simulink model "signal_tranmission"  (R2024b)
settings: Solver=ode45  StartTime=0.0  StopTime=10  FixedStep=0.000125  RelTol=1e-3
libraries: dspfdesign x500, commchan3 x1
(part 5 of 7)

== system signal_tranmission/SSB Demod55/Balanced Modulator1 ==
  note: -S2(t)
  note: S1(t)
  note: -m(t)
  note: m(t)
  note: S2(t)
  note: S1(t)
  Input Signal : Inport
  Carrier Signal : Inport  Port=2
  -S2(t) : Product
  Add : Sum
  Add1 : Sum
  Add2 : Sum
  Constant : Constant
  Constant1 : Constant  Value=-1
  Constant2 : Constant
  Constant3 : Constant  Value=-1
  Product1 : Product
  S1(t) : Product
  S2(t) : Product
  DSBSC : Outport
  wires:
  Product1/1 -> Add1/1
  Add/1 -> S1(t)/1
  Constant3/1 -> -S2(t)/2
  Constant2/1 -> Add1/2
  S2(t)/1 -> -S2(t)/1
  Carrier Signal/1 -> S1(t)/2, S2(t)/1
  Constant/1 -> Add/2
  Add1/1 -> S2(t)/2
  Constant1/1 -> Product1/2
  -S2(t)/1 -> Add2/2
  S1(t)/1 -> Add2/1
  Input Signal/1 -> Product1/1, Add/1
  Add2/1 -> DSBSC/1

== system signal_tranmission/SSB Demod56/Balanced Modulator1 ==
  note: -S2(t)
  note: S1(t)
  note: -m(t)
  note: m(t)
  note: S2(t)
  note: S1(t)
  Input Signal : Inport
  Carrier Signal : Inport  Port=2
  -S2(t) : Product
  Add : Sum
  Add1 : Sum
  Add2 : Sum
  Constant : Constant
  Constant1 : Constant  Value=-1
  Constant2 : Constant
  Constant3 : Constant  Value=-1
  Product1 : Product
  S1(t) : Product
  S2(t) : Product
  DSBSC : Outport
  wires:
  Product1/1 -> Add1/1
  Add/1 -> S1(t)/1
  Constant3/1 -> -S2(t)/2
  Constant2/1 -> Add1/2
  S2(t)/1 -> -S2(t)/1
  Carrier Signal/1 -> S1(t)/2, S2(t)/1
  Constant/1 -> Add/2
  Add1/1 -> S2(t)/2
  Constant1/1 -> Product1/2
  -S2(t)/1 -> Add2/2
  S1(t)/1 -> Add2/1
  Input Signal/1 -> Product1/1, Add/1
  Add2/1 -> DSBSC/1

== system signal_tranmission/SSB Demod57/Balanced Modulator1 ==
  note: -S2(t)
  note: S1(t)
  note: -m(t)
  note: m(t)
  note: S2(t)
  note: S1(t)
  Input Signal : Inport
  Carrier Signal : Inport  Port=2
  -S2(t) : Product
  Add : Sum
  Add1 : Sum
  Add2 : Sum
  Constant : Constant
  Constant1 : Constant  Value=-1
  Constant2 : Constant
  Constant3 : Constant  Value=-1
  Product1 : Product
  S1(t) : Product
  S2(t) : Product
  DSBSC : Outport
  wires:
  Product1/1 -> Add1/1
  Add/1 -> S1(t)/1
  Constant3/1 -> -S2(t)/2
  Constant2/1 -> Add1/2
  S2(t)/1 -> -S2(t)/1
  Carrier Signal/1 -> S1(t)/2, S2(t)/1
  Constant/1 -> Add/2
  Add1/1 -> S2(t)/2
  Constant1/1 -> Product1/2
  -S2(t)/1 -> Add2/2
  S1(t)/1 -> Add2/1
  Input Signal/1 -> Product1/1, Add/1
  Add2/1 -> DSBSC/1

== system signal_tranmission/SSB Demod58/Balanced Modulator1 ==
  note: -S2(t)
  note: S1(t)
  note: -m(t)
  note: m(t)
  note: S2(t)
  note: S1(t)
  Input Signal : Inport
  Carrier Signal : Inport  Port=2
  -S2(t) : Product
  Add : Sum
  Add1 : Sum
  Add2 : Sum
  Constant : Constant
  Constant1 : Constant  Value=-1
  Constant2 : Constant
  Constant3 : Constant  Value=-1
  Product1 : Product
  S1(t) : Product
  S2(t) : Product
  DSBSC : Outport
  wires:
  Product1/1 -> Add1/1
  Add/1 -> S1(t)/1
  Constant3/1 -> -S2(t)/2
  Constant2/1 -> Add1/2
  S2(t)/1 -> -S2(t)/1
  Carrier Signal/1 -> S1(t)/2, S2(t)/1
  Constant/1 -> Add/2
  Add1/1 -> S2(t)/2
  Constant1/1 -> Product1/2
  -S2(t)/1 -> Add2/2
  S1(t)/1 -> Add2/1
  Input Signal/1 -> Product1/1, Add/1
  Add2/1 -> DSBSC/1

== system signal_tranmission/SSB Demod59/Balanced Modulator1 ==
  note: -S2(t)
  note: S1(t)
  note: -m(t)
  note: m(t)
  note: S2(t)
  note: S1(t)
  Input Signal : Inport
  Carrier Signal : Inport  Port=2
  -S2(t) : Product
  Add : Sum
  Add1 : Sum
  Add2 : Sum
  Constant : Constant
  Constant1 : Constant  Value=-1
  Constant2 : Constant
  Constant3 : Constant  Value=-1
  Product1 : Product
  S1(t) : Product
  S2(t) : Product
  DSBSC : Outport
  wires:
  Product1/1 -> Add1/1
  Add/1 -> S1(t)/1
  Constant3/1 -> -S2(t)/2
  Constant2/1 -> Add1/2
  S2(t)/1 -> -S2(t)/1
  Carrier Signal/1 -> S1(t)/2, S2(t)/1
  Constant/1 -> Add/2
  Add1/1 -> S2(t)/2
  Constant1/1 -> Product1/2
  -S2(t)/1 -> Add2/2
  S1(t)/1 -> Add2/1
  Input Signal/1 -> Product1/1, Add/1
  Add2/1 -> DSBSC/1

== system signal_tranmission/SSB Demod6/Balanced Modulator1 ==
  note: -S2(t)
  note: S1(t)
  note: -m(t)
  note: m(t)
  note: S2(t)
  note: S1(t)
  Input Signal : Inport
  Carrier Signal : Inport  Port=2
  -S2(t) : Product
  Add : Sum
  Add1 : Sum
  Add2 : Sum
  Constant : Constant
  Constant1 : Constant  Value=-1
  Constant2 : Constant
  Constant3 : Constant  Value=-1
  Product1 : Product
  S1(t) : Product
  S2(t) : Product
  DSBSC : Outport
  wires:
  Product1/1 -> Add1/1
  Add/1 -> S1(t)/1
  Constant3/1 -> -S2(t)/2
  Constant2/1 -> Add1/2
  S2(t)/1 -> -S2(t)/1
  Carrier Signal/1 -> S1(t)/2, S2(t)/1
  Constant/1 -> Add/2
  Add1/1 -> S2(t)/2
  Constant1/1 -> Product1/2
  -S2(t)/1 -> Add2/2
  S1(t)/1 -> Add2/1
  Input Signal/1 -> Product1/1, Add/1
  Add2/1 -> DSBSC/1

== system signal_tranmission/SSB Demod60/Balanced Modulator1 ==
  note: -S2(t)
  note: S1(t)
  note: -m(t)
  note: m(t)
  note: S2(t)
  note: S1(t)
  Input Signal : Inport
  Carrier Signal : Inport  Port=2
  -S2(t) : Product
  Add : Sum
  Add1 : Sum
  Add2 : Sum
  Constant : Constant
  Constant1 : Constant  Value=-1
  Constant2 : Constant
  Constant3 : Constant  Value=-1
  Product1 : Product
  S1(t) : Product
  S2(t) : Product
  DSBSC : Outport
  wires:
  Product1/1 -> Add1/1
  Add/1 -> S1(t)/1
  Constant3/1 -> -S2(t)/2
  Constant2/1 -> Add1/2
  S2(t)/1 -> -S2(t)/1
  Carrier Signal/1 -> S1(t)/2, S2(t)/1
  Constant/1 -> Add/2
  Add1/1 -> S2(t)/2
  Constant1/1 -> Product1/2
  -S2(t)/1 -> Add2/2
  S1(t)/1 -> Add2/1
  Input Signal/1 -> Product1/1, Add/1
  Add2/1 -> DSBSC/1

== system signal_tranmission/SSB Demod61/Balanced Modulator1 ==
  note: -S2(t)
  note: S1(t)
  note: -m(t)
  note: m(t)
  note: S2(t)
  note: S1(t)
  Input Signal : Inport
  Carrier Signal : Inport  Port=2
  -S2(t) : Product
  Add : Sum
  Add1 : Sum
  Add2 : Sum
  Constant : Constant
  Constant1 : Constant  Value=-1
  Constant2 : Constant
  Constant3 : Constant  Value=-1
  Product1 : Product
  S1(t) : Product
  S2(t) : Product
  DSBSC : Outport
  wires:
  Product1/1 -> Add1/1
  Add/1 -> S1(t)/1
  Constant3/1 -> -S2(t)/2
  Constant2/1 -> Add1/2
  S2(t)/1 -> -S2(t)/1
  Carrier Signal/1 -> S1(t)/2, S2(t)/1
  Constant/1 -> Add/2
  Add1/1 -> S2(t)/2
  Constant1/1 -> Product1/2
  -S2(t)/1 -> Add2/2
  S1(t)/1 -> Add2/1
  Input Signal/1 -> Product1/1, Add/1
  Add2/1 -> DSBSC/1

== system signal_tranmission/SSB Demod62/Balanced Modulator1 ==
  note: -S2(t)
  note: S1(t)
  note: -m(t)
  note: m(t)
  note: S2(t)
  note: S1(t)
  Input Signal : Inport
  Carrier Signal : Inport  Port=2
  -S2(t) : Product
  Add : Sum
  Add1 : Sum
  Add2 : Sum
  Constant : Constant
  Constant1 : Constant  Value=-1
  Constant2 : Constant
  Constant3 : Constant  Value=-1
  Product1 : Product
  S1(t) : Product
  S2(t) : Product
  DSBSC : Outport
  wires:
  Product1/1 -> Add1/1
  Add/1 -> S1(t)/1
  Constant3/1 -> -S2(t)/2
  Constant2/1 -> Add1/2
  S2(t)/1 -> -S2(t)/1
  Carrier Signal/1 -> S1(t)/2, S2(t)/1
  Constant/1 -> Add/2
  Add1/1 -> S2(t)/2
  Constant1/1 -> Product1/2
  -S2(t)/1 -> Add2/2
  S1(t)/1 -> Add2/1
  Input Signal/1 -> Product1/1, Add/1
  Add2/1 -> DSBSC/1

== system signal_tranmission/SSB Demod63/Balanced Modulator1 ==
  note: -S2(t)
  note: S1(t)
  note: -m(t)
  note: m(t)
  note: S2(t)
  note: S1(t)
  Input Signal : Inport
  Carrier Signal : Inport  Port=2
  -S2(t) : Product
  Add : Sum
  Add1 : Sum
  Add2 : Sum
  Constant : Constant
  Constant1 : Constant  Value=-1
  Constant2 : Constant
  Constant3 : Constant  Value=-1
  Product1 : Product
  S1(t) : Product
  S2(t) : Product
  DSBSC : Outport
  wires:
  Product1/1 -> Add1/1
  Add/1 -> S1(t)/1
  Constant3/1 -> -S2(t)/2
  Constant2/1 -> Add1/2
  S2(t)/1 -> -S2(t)/1
  Carrier Signal/1 -> S1(t)/2, S2(t)/1
  Constant/1 -> Add/2
  Add1/1 -> S2(t)/2
  Constant1/1 -> Product1/2
  -S2(t)/1 -> Add2/2
  S1(t)/1 -> Add2/1
  Input Signal/1 -> Product1/1, Add/1
  Add2/1 -> DSBSC/1

== system signal_tranmission/SSB Demod64/Balanced Modulator1 ==
  note: -S2(t)
  note: S1(t)
  note: -m(t)
  note: m(t)
  note: S2(t)
  note: S1(t)
  Input Signal : Inport
  Carrier Signal : Inport  Port=2
  -S2(t) : Product
  Add : Sum
  Add1 : Sum
  Add2 : Sum
  Constant : Constant
  Constant1 : Constant  Value=-1
  Constant2 : Constant
  Constant3 : Constant  Value=-1
  Product1 : Product
  S1(t) : Product
  S2(t) : Product
  DSBSC : Outport
  wires:
  Product1/1 -> Add1/1
  Add/1 -> S1(t)/1
  Constant3/1 -> -S2(t)/2
  Constant2/1 -> Add1/2
  S2(t)/1 -> -S2(t)/1
  Carrier Signal/1 -> S1(t)/2, S2(t)/1
  Constant/1 -> Add/2
  Add1/1 -> S2(t)/2
  Constant1/1 -> Product1/2
  -S2(t)/1 -> Add2/2
  S1(t)/1 -> Add2/1
  Input Signal/1 -> Product1/1, Add/1
  Add2/1 -> DSBSC/1

== system signal_tranmission/SSB Demod65/Balanced Modulator1 ==
  note: -S2(t)
  note: S1(t)
  note: -m(t)
  note: m(t)
  note: S2(t)
  note: S1(t)
  Input Signal : Inport
  Carrier Signal : Inport  Port=2
  -S2(t) : Product
  Add : Sum
  Add1 : Sum
  Add2 : Sum
  Constant : Constant
  Constant1 : Constant  Value=-1
  Constant2 : Constant
  Constant3 : Constant  Value=-1
  Product1 : Product
  S1(t) : Product
  S2(t) : Product
  DSBSC : Outport
  wires:
  Product1/1 -> Add1/1
  Add/1 -> S1(t)/1
  Constant3/1 -> -S2(t)/2
  Constant2/1 -> Add1/2
  S2(t)/1 -> -S2(t)/1
  Carrier Signal/1 -> S1(t)/2, S2(t)/1
  Constant/1 -> Add/2
  Add1/1 -> S2(t)/2
  Constant1/1 -> Product1/2
  -S2(t)/1 -> Add2/2
  S1(t)/1 -> Add2/1
  Input Signal/1 -> Product1/1, Add/1
  Add2/1 -> DSBSC/1

== system signal_tranmission/SSB Demod66/Balanced Modulator1 ==
  note: -S2(t)
  note: S1(t)
  note: -m(t)
  note: m(t)
  note: S2(t)
  note: S1(t)
  Input Signal : Inport
  Carrier Signal : Inport  Port=2
  -S2(t) : Product
  Add : Sum
  Add1 : Sum
  Add2 : Sum
  Constant : Constant
  Constant1 : Constant  Value=-1
  Constant2 : Constant
  Constant3 : Constant  Value=-1
  Product1 : Product
  S1(t) : Product
  S2(t) : Product
  DSBSC : Outport
  wires:
  Product1/1 -> Add1/1
  Add/1 -> S1(t)/1
  Constant3/1 -> -S2(t)/2
  Constant2/1 -> Add1/2
  S2(t)/1 -> -S2(t)/1
  Carrier Signal/1 -> S1(t)/2, S2(t)/1
  Constant/1 -> Add/2
  Add1/1 -> S2(t)/2
  Constant1/1 -> Product1/2
  -S2(t)/1 -> Add2/2
  S1(t)/1 -> Add2/1
  Input Signal/1 -> Product1/1, Add/1
  Add2/1 -> DSBSC/1

== system signal_tranmission/SSB Demod67/Balanced Modulator1 ==
  note: -S2(t)
  note: S1(t)
  note: -m(t)
  note: m(t)
  note: S2(t)
  note: S1(t)
  Input Signal : Inport
  Carrier Signal : Inport  Port=2
  -S2(t) : Product
  Add : Sum
  Add1 : Sum
  Add2 : Sum
  Constant : Constant
  Constant1 : Constant  Value=-1
  Constant2 : Constant
  Constant3 : Constant  Value=-1
  Product1 : Product
  S1(t) : Product
  S2(t) : Product
  DSBSC : Outport
  wires:
  Product1/1 -> Add1/1
  Add/1 -> S1(t)/1
  Constant3/1 -> -S2(t)/2
  Constant2/1 -> Add1/2
  S2(t)/1 -> -S2(t)/1
  Carrier Signal/1 -> S1(t)/2, S2(t)/1
  Constant/1 -> Add/2
  Add1/1 -> S2(t)/2
  Constant1/1 -> Product1/2
  -S2(t)/1 -> Add2/2
  S1(t)/1 -> Add2/1
  Input Signal/1 -> Product1/1, Add/1
  Add2/1 -> DSBSC/1

== system signal_tranmission/SSB Demod68/Balanced Modulator1 ==
  note: -S2(t)
  note: S1(t)
  note: -m(t)
  note: m(t)
  note: S2(t)
  note: S1(t)
  Input Signal : Inport
  Carrier Signal : Inport  Port=2
  -S2(t) : Product
  Add : Sum
  Add1 : Sum
  Add2 : Sum
  Constant : Constant
  Constant1 : Constant  Value=-1
  Constant2 : Constant
  Constant3 : Constant  Value=-1
  Product1 : Product
  S1(t) : Product
  S2(t) : Product
  DSBSC : Outport
  wires:
  Product1/1 -> Add1/1
  Add/1 -> S1(t)/1
  Constant3/1 -> -S2(t)/2
  Constant2/1 -> Add1/2
  S2(t)/1 -> -S2(t)/1
  Carrier Signal/1 -> S1(t)/2, S2(t)/1
  Constant/1 -> Add/2
  Add1/1 -> S2(t)/2
  Constant1/1 -> Product1/2
  -S2(t)/1 -> Add2/2
  S1(t)/1 -> Add2/1
  Input Signal/1 -> Product1/1, Add/1
  Add2/1 -> DSBSC/1

== system signal_tranmission/SSB Demod69/Balanced Modulator1 ==
  note: -S2(t)
  note: S1(t)
  note: -m(t)
  note: m(t)
  note: S2(t)
  note: S1(t)
  Input Signal : Inport
  Carrier Signal : Inport  Port=2
  -S2(t) : Product
  Add : Sum
  Add1 : Sum
  Add2 : Sum
  Constant : Constant
  Constant1 : Constant  Value=-1
  Constant2 : Constant
  Constant3 : Constant  Value=-1
  Product1 : Product
  S1(t) : Product
  S2(t) : Product
  DSBSC : Outport
  wires:
  Product1/1 -> Add1/1
  Add/1 -> S1(t)/1
  Constant3/1 -> -S2(t)/2
  Constant2/1 -> Add1/2
  S2(t)/1 -> -S2(t)/1
  Carrier Signal/1 -> S1(t)/2, S2(t)/1
  Constant/1 -> Add/2
  Add1/1 -> S2(t)/2
  Constant1/1 -> Product1/2
  -S2(t)/1 -> Add2/2
  S1(t)/1 -> Add2/1
  Input Signal/1 -> Product1/1, Add/1
  Add2/1 -> DSBSC/1

== system signal_tranmission/SSB Demod7/Balanced Modulator1 ==
  note: -S2(t)
  note: S1(t)
  note: -m(t)
  note: m(t)
  note: S2(t)
  note: S1(t)
  Input Signal : Inport
  Carrier Signal : Inport  Port=2
  -S2(t) : Product
  Add : Sum
  Add1 : Sum
  Add2 : Sum
  Constant : Constant
  Constant1 : Constant  Value=-1
  Constant2 : Constant
  Constant3 : Constant  Value=-1
  Product1 : Product
  S1(t) : Product
  S2(t) : Product
  DSBSC : Outport
  wires:
  Product1/1 -> Add1/1
  Add/1 -> S1(t)/1
  Constant3/1 -> -S2(t)/2
  Constant2/1 -> Add1/2
  S2(t)/1 -> -S2(t)/1
  Carrier Signal/1 -> S1(t)/2, S2(t)/1
  Constant/1 -> Add/2
  Add1/1 -> S2(t)/2
  Constant1/1 -> Product1/2
  -S2(t)/1 -> Add2/2
  S1(t)/1 -> Add2/1
  Input Signal/1 -> Product1/1, Add/1
  Add2/1 -> DSBSC/1

== system signal_tranmission/SSB Demod70/Balanced Modulator1 ==
  note: -S2(t)
  note: S1(t)
  note: -m(t)
  note: m(t)
  note: S2(t)
  note: S1(t)
  Input Signal : Inport
  Carrier Signal : Inport  Port=2
  -S2(t) : Product
  Add : Sum
  Add1 : Sum
  Add2 : Sum
  Constant : Constant
  Constant1 : Constant  Value=-1
  Constant2 : Constant
  Constant3 : Constant  Value=-1
  Product1 : Product
  S1(t) : Product
  S2(t) : Product
  DSBSC : Outport
  wires:
  Product1/1 -> Add1/1
  Add/1 -> S1(t)/1
  Constant3/1 -> -S2(t)/2
  Constant2/1 -> Add1/2
  S2(t)/1 -> -S2(t)/1
  Carrier Signal/1 -> S1(t)/2, S2(t)/1
  Constant/1 -> Add/2
  Add1/1 -> S2(t)/2
  Constant1/1 -> Product1/2
  -S2(t)/1 -> Add2/2
  S1(t)/1 -> Add2/1
  Input Signal/1 -> Product1/1, Add/1
  Add2/1 -> DSBSC/1

== system signal_tranmission/SSB Demod71/Balanced Modulator1 ==
  note: -S2(t)
  note: S1(t)
  note: -m(t)
  note: m(t)
  note: S2(t)
  note: S1(t)
  Input Signal : Inport
  Carrier Signal : Inport  Port=2
  -S2(t) : Product
  Add : Sum
  Add1 : Sum
  Add2 : Sum
  Constant : Constant
  Constant1 : Constant  Value=-1
  Constant2 : Constant
  Constant3 : Constant  Value=-1
  Product1 : Product
  S1(t) : Product
  S2(t) : Product
  DSBSC : Outport
  wires:
  Product1/1 -> Add1/1
  Add/1 -> S1(t)/1
  Constant3/1 -> -S2(t)/2
  Constant2/1 -> Add1/2
  S2(t)/1 -> -S2(t)/1
  Carrier Signal/1 -> S1(t)/2, S2(t)/1
  Constant/1 -> Add/2
  Add1/1 -> S2(t)/2
  Constant1/1 -> Product1/2
  -S2(t)/1 -> Add2/2
  S1(t)/1 -> Add2/1
  Input Signal/1 -> Product1/1, Add/1
  Add2/1 -> DSBSC/1

== system signal_tranmission/SSB Demod72/Balanced Modulator1 ==
  note: -S2(t)
  note: S1(t)
  note: -m(t)
  note: m(t)
  note: S2(t)
  note: S1(t)
  Input Signal : Inport
  Carrier Signal : Inport  Port=2
  -S2(t) : Product
  Add : Sum
  Add1 : Sum
  Add2 : Sum
  Constant : Constant
  Constant1 : Constant  Value=-1
  Constant2 : Constant
  Constant3 : Constant  Value=-1
  Product1 : Product
  S1(t) : Product
  S2(t) : Product
  DSBSC : Outport
  wires:
  Product1/1 -> Add1/1
  Add/1 -> S1(t)/1
  Constant3/1 -> -S2(t)/2
  Constant2/1 -> Add1/2
  S2(t)/1 -> -S2(t)/1
  Carrier Signal/1 -> S1(t)/2, S2(t)/1
  Constant/1 -> Add/2
  Add1/1 -> S2(t)/2
  Constant1/1 -> Product1/2
  -S2(t)/1 -> Add2/2
  S1(t)/1 -> Add2/1
  Input Signal/1 -> Product1/1, Add/1
  Add2/1 -> DSBSC/1

== system signal_tranmission/SSB Demod73/Balanced Modulator1 ==
  note: -S2(t)
  note: S1(t)
  note: -m(t)
  note: m(t)
  note: S2(t)
  note: S1(t)
  Input Signal : Inport
  Carrier Signal : Inport  Port=2
  -S2(t) : Product
  Add : Sum
  Add1 : Sum
  Add2 : Sum
  Constant : Constant
  Constant1 : Constant  Value=-1
  Constant2 : Constant
  Constant3 : Constant  Value=-1
  Product1 : Product
  S1(t) : Product
  S2(t) : Product
  DSBSC : Outport
  wires:
  Product1/1 -> Add1/1
  Add/1 -> S1(t)/1
  Constant3/1 -> -S2(t)/2
  Constant2/1 -> Add1/2
  S2(t)/1 -> -S2(t)/1
  Carrier Signal/1 -> S1(t)/2, S2(t)/1
  Constant/1 -> Add/2
  Add1/1 -> S2(t)/2
  Constant1/1 -> Product1/2
  -S2(t)/1 -> Add2/2
  S1(t)/1 -> Add2/1
  Input Signal/1 -> Product1/1, Add/1
  Add2/1 -> DSBSC/1

== system signal_tranmission/SSB Demod74/Balanced Modulator1 ==
  note: -S2(t)
  note: S1(t)
  note: -m(t)
  note: m(t)
  note: S2(t)
  note: S1(t)
  Input Signal : Inport
  Carrier Signal : Inport  Port=2
  -S2(t) : Product
  Add : Sum
  Add1 : Sum
  Add2 : Sum
  Constant : Constant
  Constant1 : Constant  Value=-1
  Constant2 : Constant
  Constant3 : Constant  Value=-1
  Product1 : Product
  S1(t) : Product
  S2(t) : Product
  DSBSC : Outport
  wires:
  Product1/1 -> Add1/1
  Add/1 -> S1(t)/1
  Constant3/1 -> -S2(t)/2
  Constant2/1 -> Add1/2
  S2(t)/1 -> -S2(t)/1
  Carrier Signal/1 -> S1(t)/2, S2(t)/1
  Constant/1 -> Add/2
  Add1/1 -> S2(t)/2
  Constant1/1 -> Product1/2
  -S2(t)/1 -> Add2/2
  S1(t)/1 -> Add2/1
  Input Signal/1 -> Product1/1, Add/1
  Add2/1 -> DSBSC/1

== system signal_tranmission/SSB Demod75/Balanced Modulator1 ==
  note: -S2(t)
  note: S1(t)
  note: -m(t)
  note: m(t)
  note: S2(t)
  note: S1(t)
  Input Signal : Inport
  Carrier Signal : Inport  Port=2
  -S2(t) : Product
  Add : Sum
  Add1 : Sum
  Add2 : Sum
  Constant : Constant
  Constant1 : Constant  Value=-1
  Constant2 : Constant
  Constant3 : Constant  Value=-1
  Product1 : Product
  S1(t) : Product
  S2(t) : Product
  DSBSC : Outport
  wires:
  Product1/1 -> Add1/1
  Add/1 -> S1(t)/1
  Constant3/1 -> -S2(t)/2
  Constant2/1 -> Add1/2
  S2(t)/1 -> -S2(t)/1
  Carrier Signal/1 -> S1(t)/2, S2(t)/1
  Constant/1 -> Add/2
  Add1/1 -> S2(t)/2
  Constant1/1 -> Product1/2
  -S2(t)/1 -> Add2/2
  S1(t)/1 -> Add2/1
  Input Signal/1 -> Product1/1, Add/1
  Add2/1 -> DSBSC/1

== system signal_tranmission/SSB Demod76/Balanced Modulator1 ==
  note: -S2(t)
  note: S1(t)
  note: -m(t)
  note: m(t)
  note: S2(t)
  note: S1(t)
  Input Signal : Inport
  Carrier Signal : Inport  Port=2
  -S2(t) : Product
  Add : Sum
  Add1 : Sum
  Add2 : Sum
  Constant : Constant
  Constant1 : Constant  Value=-1
  Constant2 : Constant
  Constant3 : Constant  Value=-1
  Product1 : Product
  S1(t) : Product
  S2(t) : Product
  DSBSC : Outport
  wires:
  Product1/1 -> Add1/1
  Add/1 -> S1(t)/1
  Constant3/1 -> -S2(t)/2
  Constant2/1 -> Add1/2
  S2(t)/1 -> -S2(t)/1
  Carrier Signal/1 -> S1(t)/2, S2(t)/1
  Constant/1 -> Add/2
  Add1/1 -> S2(t)/2
  Constant1/1 -> Product1/2
  -S2(t)/1 -> Add2/2
  S1(t)/1 -> Add2/1
  Input Signal/1 -> Product1/1, Add/1
  Add2/1 -> DSBSC/1

== system signal_tranmission/SSB Demod77/Balanced Modulator1 ==
  note: -S2(t)
  note: S1(t)
  note: -m(t)
  note: m(t)
  note: S2(t)
  note: S1(t)
  Input Signal : Inport
  Carrier Signal : Inport  Port=2
  -S2(t) : Product
  Add : Sum
  Add1 : Sum
  Add2 : Sum
  Constant : Constant
  Constant1 : Constant  Value=-1
  Constant2 : Constant
  Constant3 : Constant  Value=-1
  Product1 : Product
  S1(t) : Product
  S2(t) : Product
  DSBSC : Outport
  wires:
  Product1/1 -> Add1/1
  Add/1 -> S1(t)/1
  Constant3/1 -> -S2(t)/2
  Constant2/1 -> Add1/2
  S2(t)/1 -> -S2(t)/1
  Carrier Signal/1 -> S1(t)/2, S2(t)/1
  Constant/1 -> Add/2
  Add1/1 -> S2(t)/2
  Constant1/1 -> Product1/2
  -S2(t)/1 -> Add2/2
  S1(t)/1 -> Add2/1
  Input Signal/1 -> Product1/1, Add/1
  Add2/1 -> DSBSC/1

== system signal_tranmission/SSB Demod78/Balanced Modulator1 ==
  note: -S2(t)
  note: S1(t)
  note: -m(t)
  note: m(t)
  note: S2(t)
  note: S1(t)
  Input Signal : Inport
  Carrier Signal : Inport  Port=2
  -S2(t) : Product
  Add : Sum
  Add1 : Sum
  Add2 : Sum
  Constant : Constant
  Constant1 : Constant  Value=-1
  Constant2 : Constant
  Constant3 : Constant  Value=-1
  Product1 : Product
  S1(t) : Product
  S2(t) : Product
  DSBSC : Outport
  wires:
  Product1/1 -> Add1/1
  Add/1 -> S1(t)/1
  Constant3/1 -> -S2(t)/2
  Constant2/1 -> Add1/2
  S2(t)/1 -> -S2(t)/1
  Carrier Signal/1 -> S1(t)/2, S2(t)/1
  Constant/1 -> Add/2
  Add1/1 -> S2(t)/2
  Constant1/1 -> Product1/2
  -S2(t)/1 -> Add2/2
  S1(t)/1 -> Add2/1
  Input Signal/1 -> Product1/1, Add/1
  Add2/1 -> DSBSC/1

== system signal_tranmission/SSB Demod79/Balanced Modulator1 ==
  note: -S2(t)
  note: S1(t)
  note: -m(t)
  note: m(t)
  note: S2(t)
  note: S1(t)
  Input Signal : Inport
  Carrier Signal : Inport  Port=2
  -S2(t) : Product
  Add : Sum
  Add1 : Sum
  Add2 : Sum
  Constant : Constant
  Constant1 : Constant  Value=-1
  Constant2 : Constant
  Constant3 : Constant  Value=-1
  Product1 : Product
  S1(t) : Product
  S2(t) : Product
  DSBSC : Outport
  wires:
  Product1/1 -> Add1/1
  Add/1 -> S1(t)/1
  Constant3/1 -> -S2(t)/2
  Constant2/1 -> Add1/2
  S2(t)/1 -> -S2(t)/1
  Carrier Signal/1 -> S1(t)/2, S2(t)/1
  Constant/1 -> Add/2
  Add1/1 -> S2(t)/2
  Constant1/1 -> Product1/2
  -S2(t)/1 -> Add2/2
  S1(t)/1 -> Add2/1
  Input Signal/1 -> Product1/1, Add/1
  Add2/1 -> DSBSC/1

== system signal_tranmission/SSB Demod8/Balanced Modulator1 ==
  note: -S2(t)
  note: S1(t)
  note: -m(t)
  note: m(t)
  note: S2(t)
  note: S1(t)
  Input Signal : Inport
  Carrier Signal : Inport  Port=2
  -S2(t) : Product
  Add : Sum
  Add1 : Sum
  Add2 : Sum
  Constant : Constant
  Constant1 : Constant  Value=-1
  Constant2 : Constant
  Constant3 : Constant  Value=-1
  Product1 : Product
  S1(t) : Product
  S2(t) : Product
  DSBSC : Outport
  wires:
  Product1/1 -> Add1/1
  Add/1 -> S1(t)/1
  Constant3/1 -> -S2(t)/2
  Constant2/1 -> Add1/2
  S2(t)/1 -> -S2(t)/1
  Carrier Signal/1 -> S1(t)/2, S2(t)/1
  Constant/1 -> Add/2
  Add1/1 -> S2(t)/2
  Constant1/1 -> Product1/2
  -S2(t)/1 -> Add2/2
  S1(t)/1 -> Add2/1
  Input Signal/1 -> Product1/1, Add/1
  Add2/1 -> DSBSC/1

== system signal_tranmission/SSB Demod80/Balanced Modulator1 ==
  note: -S2(t)
  note: S1(t)
  note: -m(t)
  note: m(t)
  note: S2(t)
  note: S1(t)
  Input Signal : Inport
  Carrier Signal : Inport  Port=2
  -S2(t) : Product
  Add : Sum
  Add1 : Sum
  Add2 : Sum
  Constant : Constant
  Constant1 : Constant  Value=-1
  Constant2 : Constant
  Constant3 : Constant  Value=-1
  Product1 : Product
  S1(t) : Product
  S2(t) : Product
  DSBSC : Outport
  wires:
  Product1/1 -> Add1/1
  Add/1 -> S1(t)/1
  Constant3/1 -> -S2(t)/2
  Constant2/1 -> Add1/2
  S2(t)/1 -> -S2(t)/1
  Carrier Signal/1 -> S1(t)/2, S2(t)/1
  Constant/1 -> Add/2
  Add1/1 -> S2(t)/2
  Constant1/1 -> Product1/2
  -S2(t)/1 -> Add2/2
  S1(t)/1 -> Add2/1
  Input Signal/1 -> Product1/1, Add/1
  Add2/1 -> DSBSC/1

== system signal_tranmission/SSB Demod81/Balanced Modulator1 ==
  note: -S2(t)
  note: S1(t)
  note: -m(t)
  note: m(t)
  note: S2(t)
  note: S1(t)
  Input Signal : Inport
  Carrier Signal : Inport  Port=2
  -S2(t) : Product
  Add : Sum
  Add1 : Sum
  Add2 : Sum
  Constant : Constant
  Constant1 : Constant  Value=-1
  Constant2 : Constant
  Constant3 : Constant  Value=-1
  Product1 : Product
  S1(t) : Product
  S2(t) : Product
  DSBSC : Outport
  wires:
  Product1/1 -> Add1/1
  Add/1 -> S1(t)/1
  Constant3/1 -> -S2(t)/2
  Constant2/1 -> Add1/2
  S2(t)/1 -> -S2(t)/1
  Carrier Signal/1 -> S1(t)/2, S2(t)/1
  Constant/1 -> Add/2
  Add1/1 -> S2(t)/2
  Constant1/1 -> Product1/2
  -S2(t)/1 -> Add2/2
  S1(t)/1 -> Add2/1
  Input Signal/1 -> Product1/1, Add/1
  Add2/1 -> DSBSC/1

== system signal_tranmission/SSB Demod82/Balanced Modulator1 ==
  note: -S2(t)
  note: S1(t)
  note: -m(t)
  note: m(t)
  note: S2(t)
  note: S1(t)
  Input Signal : Inport
  Carrier Signal : Inport  Port=2
  -S2(t) : Product
  Add : Sum
  Add1 : Sum
  Add2 : Sum
  Constant : Constant
  Constant1 : Constant  Value=-1
  Constant2 : Constant
  Constant3 : Constant  Value=-1
  Product1 : Product
  S1(t) : Product
  S2(t) : Product
  DSBSC : Outport
  wires:
  Product1/1 -> Add1/1
  Add/1 -> S1(t)/1
  Constant3/1 -> -S2(t)/2
  Constant2/1 -> Add1/2
  S2(t)/1 -> -S2(t)/1
  Carrier Signal/1 -> S1(t)/2, S2(t)/1
  Constant/1 -> Add/2
  Add1/1 -> S2(t)/2
  Constant1/1 -> Product1/2
  -S2(t)/1 -> Add2/2
  S1(t)/1 -> Add2/1
  Input Signal/1 -> Product1/1, Add/1
  Add2/1 -> DSBSC/1

== system signal_tranmission/SSB Demod83/Balanced Modulator1 ==
  note: -S2(t)
  note: S1(t)
  note: -m(t)
  note: m(t)
  note: S2(t)
  note: S1(t)
  Input Signal : Inport
  Carrier Signal : Inport  Port=2
  -S2(t) : Product
  Add : Sum
  Add1 : Sum
  Add2 : Sum
  Constant : Constant
  Constant1 : Constant  Value=-1
  Constant2 : Constant
  Constant3 : Constant  Value=-1
  Product1 : Product
  S1(t) : Product
  S2(t) : Product
  DSBSC : Outport
  wires:
  Product1/1 -> Add1/1
  Add/1 -> S1(t)/1
  Constant3/1 -> -S2(t)/2
  Constant2/1 -> Add1/2
  S2(t)/1 -> -S2(t)/1
  Carrier Signal/1 -> S1(t)/2, S2(t)/1
  Constant/1 -> Add/2
  Add1/1 -> S2(t)/2
  Constant1/1 -> Product1/2
  -S2(t)/1 -> Add2/2
  S1(t)/1 -> Add2/1
  Input Signal/1 -> Product1/1, Add/1
  Add2/1 -> DSBSC/1

== system signal_tranmission/SSB Demod84/Balanced Modulator1 ==
  note: -S2(t)
  note: S1(t)
  note: -m(t)
  note: m(t)
  note: S2(t)
  note: S1(t)
  Input Signal : Inport
  Carrier Signal : Inport  Port=2
  -S2(t) : Product
  Add : Sum
  Add1 : Sum
  Add2 : Sum
  Constant : Constant
  Constant1 : Constant  Value=-1
  Constant2 : Constant
  Constant3 : Constant  Value=-1
  Product1 : Product
  S1(t) : Product
  S2(t) : Product
  DSBSC : Outport
  wires:
  Product1/1 -> Add1/1
  Add/1 -> S1(t)/1
  Constant3/1 -> -S2(t)/2
  Constant2/1 -> Add1/2
  S2(t)/1 -> -S2(t)/1
  Carrier Signal/1 -> S1(t)/2, S2(t)/1
  Constant/1 -> Add/2
  Add1/1 -> S2(t)/2
  Constant1/1 -> Product1/2
  -S2(t)/1 -> Add2/2
  S1(t)/1 -> Add2/1
  Input Signal/1 -> Product1/1, Add/1
  Add2/1 -> DSBSC/1

== system signal_tranmission/SSB Demod85/Balanced Modulator1 ==
  note: -S2(t)
  note: S1(t)
  note: -m(t)
  note: m(t)
  note: S2(t)
  note: S1(t)
  Input Signal : Inport
  Carrier Signal : Inport  Port=2
  -S2(t) : Product
  Add : Sum
  Add1 : Sum
  Add2 : Sum
  Constant : Constant
  Constant1 : Constant  Value=-1
  Constant2 : Constant
  Constant3 : Constant  Value=-1
  Product1 : Product
  S1(t) : Product
  S2(t) : Product
  DSBSC : Outport
  wires:
  Product1/1 -> Add1/1
  Add/1 -> S1(t)/1
  Constant3/1 -> -S2(t)/2
  Constant2/1 -> Add1/2
  S2(t)/1 -> -S2(t)/1
  Carrier Signal/1 -> S1(t)/2, S2(t)/1
  Constant/1 -> Add/2
  Add1/1 -> S2(t)/2
  Constant1/1 -> Product1/2
  -S2(t)/1 -> Add2/2
  S1(t)/1 -> Add2/1
  Input Signal/1 -> Product1/1, Add/1
  Add2/1 -> DSBSC/1

== system signal_tranmission/SSB Demod86/Balanced Modulator1 ==
  note: -S2(t)
  note: S1(t)
  note: -m(t)
  note: m(t)
  note: S2(t)
  note: S1(t)
  Input Signal : Inport
  Carrier Signal : Inport  Port=2
  -S2(t) : Product
  Add : Sum
  Add1 : Sum
  Add2 : Sum
  Constant : Constant
  Constant1 : Constant  Value=-1
  Constant2 : Constant
  Constant3 : Constant  Value=-1
  Product1 : Product
  S1(t) : Product
  S2(t) : Product
  DSBSC : Outport
  wires:
  Product1/1 -> Add1/1
  Add/1 -> S1(t)/1
  Constant3/1 -> -S2(t)/2
  Constant2/1 -> Add1/2
  S2(t)/1 -> -S2(t)/1
  Carrier Signal/1 -> S1(t)/2, S2(t)/1
  Constant/1 -> Add/2
  Add1/1 -> S2(t)/2
  Constant1/1 -> Product1/2
  -S2(t)/1 -> Add2/2
  S1(t)/1 -> Add2/1
  Input Signal/1 -> Product1/1, Add/1
  Add2/1 -> DSBSC/1

== system signal_tranmission/SSB Demod87/Balanced Modulator1 ==
  note: -S2(t)
  note: S1(t)
  note: -m(t)
  note: m(t)
  note: S2(t)
  note: S1(t)
  Input Signal : Inport
  Carrier Signal : Inport  Port=2
  -S2(t) : Product
  Add : Sum
  Add1 : Sum
  Add2 : Sum
  Constant : Constant
  Constant1 : Constant  Value=-1
  Constant2 : Constant
  Constant3 : Constant  Value=-1
  Product1 : Product
  S1(t) : Product
  S2(t) : Product
  DSBSC : Outport
  wires:
  Product1/1 -> Add1/1
  Add/1 -> S1(t)/1
  Constant3/1 -> -S2(t)/2
  Constant2/1 -> Add1/2
  S2(t)/1 -> -S2(t)/1
  Carrier Signal/1 -> S1(t)/2, S2(t)/1
  Constant/1 -> Add/2
  Add1/1 -> S2(t)/2
  Constant1/1 -> Product1/2
  -S2(t)/1 -> Add2/2
  S1(t)/1 -> Add2/1
  Input Signal/1 -> Product1/1, Add/1
  Add2/1 -> DSBSC/1

== system signal_tranmission/SSB Demod88/Balanced Modulator1 ==
  note: -S2(t)
  note: S1(t)
  note: -m(t)
  note: m(t)
  note: S2(t)
  note: S1(t)
  Input Signal : Inport
  Carrier Signal : Inport  Port=2
  -S2(t) : Product
  Add : Sum
  Add1 : Sum
  Add2 : Sum
  Constant : Constant
  Constant1 : Constant  Value=-1
  Constant2 : Constant
  Constant3 : Constant  Value=-1
  Product1 : Product
  S1(t) : Product
  S2(t) : Product
  DSBSC : Outport
  wires:
  Product1/1 -> Add1/1
  Add/1 -> S1(t)/1
  Constant3/1 -> -S2(t)/2
  Constant2/1 -> Add1/2
  S2(t)/1 -> -S2(t)/1
  Carrier Signal/1 -> S1(t)/2, S2(t)/1
  Constant/1 -> Add/2
  Add1/1 -> S2(t)/2
  Constant1/1 -> Product1/2
  -S2(t)/1 -> Add2/2
  S1(t)/1 -> Add2/1
  Input Signal/1 -> Product1/1, Add/1
  Add2/1 -> DSBSC/1

== system signal_tranmission/SSB Demod89/Balanced Modulator1 ==
  note: -S2(t)
  note: S1(t)
  note: -m(t)
  note: m(t)
  note: S2(t)
  note: S1(t)
  Input Signal : Inport
  Carrier Signal : Inport  Port=2
  -S2(t) : Product
  Add : Sum
  Add1 : Sum
  Add2 : Sum
  Constant : Constant
  Constant1 : Constant  Value=-1
  Constant2 : Constant
  Constant3 : Constant  Value=-1
  Product1 : Product
  S1(t) : Product
  S2(t) : Product
  DSBSC : Outport
  wires:
  Product1/1 -> Add1/1
  Add/1 -> S1(t)/1
  Constant3/1 -> -S2(t)/2
  Constant2/1 -> Add1/2
  S2(t)/1 -> -S2(t)/1
  Carrier Signal/1 -> S1(t)/2, S2(t)/1
  Constant/1 -> Add/2
  Add1/1 -> S2(t)/2
  Constant1/1 -> Product1/2
  -S2(t)/1 -> Add2/2
  S1(t)/1 -> Add2/1
  Input Signal/1 -> Product1/1, Add/1
  Add2/1 -> DSBSC/1

== system signal_tranmission/SSB Demod9/Balanced Modulator1 ==
  note: -S2(t)
  note: S1(t)
  note: -m(t)
  note: m(t)
  note: S2(t)
  note: S1(t)
  Input Signal : Inport
  Carrier Signal : Inport  Port=2
  -S2(t) : Product
  Add : Sum
  Add1 : Sum
  Add2 : Sum
  Constant : Constant
  Constant1 : Constant  Value=-1
  Constant2 : Constant
  Constant3 : Constant  Value=-1
  Product1 : Product
  S1(t) : Product
  S2(t) : Product
  DSBSC : Outport
  wires:
  Product1/1 -> Add1/1
  Add/1 -> S1(t)/1
  Constant3/1 -> -S2(t)/2
  Constant2/1 -> Add1/2
  S2(t)/1 -> -S2(t)/1
  Carrier Signal/1 -> S1(t)/2, S2(t)/1
  Constant/1 -> Add/2
  Add1/1 -> S2(t)/2
  Constant1/1 -> Product1/2
  -S2(t)/1 -> Add2/2
  S1(t)/1 -> Add2/1
  Input Signal/1 -> Product1/1, Add/1
  Add2/1 -> DSBSC/1

== system signal_tranmission/SSB Demod90/Balanced Modulator1 ==
  note: -S2(t)
  note: S1(t)
  note: -m(t)
  note: m(t)
  note: S2(t)
  note: S1(t)
  Input Signal : Inport
  Carrier Signal : Inport  Port=2
  -S2(t) : Product
  Add : Sum
  Add1 : Sum
  Add2 : Sum
  Constant : Constant
  Constant1 : Constant  Value=-1
  Constant2 : Constant
  Constant3 : Constant  Value=-1
  Product1 : Product
  S1(t) : Product
  S2(t) : Product
  DSBSC : Outport
  wires:
  Product1/1 -> Add1/1
  Add/1 -> S1(t)/1
  Constant3/1 -> -S2(t)/2
  Constant2/1 -> Add1/2
  S2(t)/1 -> -S2(t)/1
  Carrier Signal/1 -> S1(t)/2, S2(t)/1
  Constant/1 -> Add/2
  Add1/1 -> S2(t)/2
  Constant1/1 -> Product1/2
  -S2(t)/1 -> Add2/2
  S1(t)/1 -> Add2/1
  Input Signal/1 -> Product1/1, Add/1
  Add2/1 -> DSBSC/1

== system signal_tranmission/SSB Demod91/Balanced Modulator1 ==
  note: -S2(t)
  note: S1(t)
  note: -m(t)
  note: m(t)
  note: S2(t)
  note: S1(t)
  Input Signal : Inport
  Carrier Signal : Inport  Port=2
  -S2(t) : Product
  Add : Sum
  Add1 : Sum
  Add2 : Sum
  Constant : Constant
  Constant1 : Constant  Value=-1
  Constant2 : Constant
  Constant3 : Constant  Value=-1
  Product1 : Product
  S1(t) : Product
  S2(t) : Product
  DSBSC : Outport
  wires:
  Product1/1 -> Add1/1
  Add/1 -> S1(t)/1
  Constant3/1 -> -S2(t)/2
  Constant2/1 -> Add1/2
  S2(t)/1 -> -S2(t)/1
  Carrier Signal/1 -> S1(t)/2, S2(t)/1
  Constant/1 -> Add/2
  Add1/1 -> S2(t)/2
  Constant1/1 -> Product1/2
  -S2(t)/1 -> Add2/2
  S1(t)/1 -> Add2/1
  Input Signal/1 -> Product1/1, Add/1
  Add2/1 -> DSBSC/1

== system signal_tranmission/SSB Demod92/Balanced Modulator1 ==
  note: -S2(t)
  note: S1(t)
  note: -m(t)
  note: m(t)
  note: S2(t)
  note: S1(t)
  Input Signal : Inport
  Carrier Signal : Inport  Port=2
  -S2(t) : Product
  Add : Sum
  Add1 : Sum
  Add2 : Sum
  Constant : Constant
  Constant1 : Constant  Value=-1
  Constant2 : Constant
  Constant3 : Constant  Value=-1
  Product1 : Product
  S1(t) : Product
  S2(t) : Product
  DSBSC : Outport
  wires:
  Product1/1 -> Add1/1
  Add/1 -> S1(t)/1
  Constant3/1 -> -S2(t)/2
  Constant2/1 -> Add1/2
  S2(t)/1 -> -S2(t)/1
  Carrier Signal/1 -> S1(t)/2, S2(t)/1
  Constant/1 -> Add/2
  Add1/1 -> S2(t)/2
  Constant1/1 -> Product1/2
  -S2(t)/1 -> Add2/2
  S1(t)/1 -> Add2/1
  Input Signal/1 -> Product1/1, Add/1
  Add2/1 -> DSBSC/1

== system signal_tranmission/SSB Demod93/Balanced Modulator1 ==
  note: -S2(t)
  note: S1(t)
  note: -m(t)
  note: m(t)
  note: S2(t)
  note: S1(t)
  Input Signal : Inport
  Carrier Signal : Inport  Port=2
  -S2(t) : Product
  Add : Sum
  Add1 : Sum
  Add2 : Sum
  Constant : Constant
  Constant1 : Constant  Value=-1
  Constant2 : Constant
  Constant3 : Constant  Value=-1
  Product1 : Product
  S1(t) : Product
  S2(t) : Product
  DSBSC : Outport
  wires:
  Product1/1 -> Add1/1
  Add/1 -> S1(t)/1
  Constant3/1 -> -S2(t)/2
  Constant2/1 -> Add1/2
  S2(t)/1 -> -S2(t)/1
  Carrier Signal/1 -> S1(t)/2, S2(t)/1
  Constant/1 -> Add/2
  Add1/1 -> S2(t)/2
  Constant1/1 -> Product1/2
  -S2(t)/1 -> Add2/2
  S1(t)/1 -> Add2/1
  Input Signal/1 -> Product1/1, Add/1
  Add2/1 -> DSBSC/1

== system signal_tranmission/SSB Demod94/Balanced Modulator1 ==
  note: -S2(t)
  note: S1(t)
  note: -m(t)
  note: m(t)
  note: S2(t)
  note: S1(t)
  Input Signal : Inport
  Carrier Signal : Inport  Port=2
  -S2(t) : Product
  Add : Sum
  Add1 : Sum
  Add2 : Sum
  Constant : Constant
  Constant1 : Constant  Value=-1
  Constant2 : Constant
  Constant3 : Constant  Value=-1
  Product1 : Product
  S1(t) : Product
  S2(t) : Product
  DSBSC : Outport
  wires:
  Product1/1 -> Add1/1
  Add/1 -> S1(t)/1
  Constant3/1 -> -S2(t)/2
  Constant2/1 -> Add1/2
  S2(t)/1 -> -S2(t)/1
  Carrier Signal/1 -> S1(t)/2, S2(t)/1
  Constant/1 -> Add/2
  Add1/1 -> S2(t)/2
  Constant1/1 -> Product1/2
  -S2(t)/1 -> Add2/2
  S1(t)/1 -> Add2/1
  Input Signal/1 -> Product1/1, Add/1
  Add2/1 -> DSBSC/1

== system signal_tranmission/SSB Demod95/Balanced Modulator1 ==
  note: -S2(t)
  note: S1(t)
  note: -m(t)
  note: m(t)
  note: S2(t)
  note: S1(t)
  Input Signal : Inport
  Carrier Signal : Inport  Port=2
  -S2(t) : Product
  Add : Sum
  Add1 : Sum
  Add2 : Sum
  Constant : Constant
  Constant1 : Constant  Value=-1
  Constant2 : Constant
  Constant3 : Constant  Value=-1
  Product1 : Product
  S1(t) : Product
  S2(t) : Product
  DSBSC : Outport
  wires:
  Product1/1 -> Add1/1
  Add/1 -> S1(t)/1
  Constant3/1 -> -S2(t)/2
  Constant2/1 -> Add1/2
  S2(t)/1 -> -S2(t)/1
  Carrier Signal/1 -> S1(t)/2, S2(t)/1
  Constant/1 -> Add/2
  Add1/1 -> S2(t)/2
  Constant1/1 -> Product1/2
  -S2(t)/1 -> Add2/2
  S1(t)/1 -> Add2/1
  Input Signal/1 -> Product1/1, Add/1
  Add2/1 -> DSBSC/1

== system signal_tranmission/SSB Demod96/Balanced Modulator1 ==
  note: -S2(t)
  note: S1(t)
  note: -m(t)
  note: m(t)
  note: S2(t)
  note: S1(t)
  Input Signal : Inport
  Carrier Signal : Inport  Port=2
  -S2(t) : Product
  Add : Sum
  Add1 : Sum
  Add2 : Sum
  Constant : Constant
  Constant1 : Constant  Value=-1
  Constant2 : Constant
  Constant3 : Constant  Value=-1
  Product1 : Product
  S1(t) : Product
  S2(t) : Product
  DSBSC : Outport
  wires:
  Product1/1 -> Add1/1
  Add/1 -> S1(t)/1
  Constant3/1 -> -S2(t)/2
  Constant2/1 -> Add1/2
  S2(t)/1 -> -S2(t)/1
  Carrier Signal/1 -> S1(t)/2, S2(t)/1
  Constant/1 -> Add/2
  Add1/1 -> S2(t)/2
  Constant1/1 -> Product1/2
  -S2(t)/1 -> Add2/2
  S1(t)/1 -> Add2/1
  Input Signal/1 -> Product1/1, Add/1
  Add2/1 -> DSBSC/1

== system signal_tranmission/SSB Demod97/Balanced Modulator1 ==
  note: -S2(t)
  note: S1(t)
  note: -m(t)
  note: m(t)
  note: S2(t)
  note: S1(t)
  Input Signal : Inport
  Carrier Signal : Inport  Port=2
  -S2(t) : Product
  Add : Sum
  Add1 : Sum
  Add2 : Sum
  Constant : Constant
  Constant1 : Constant  Value=-1
  Constant2 : Constant
  Constant3 : Constant  Value=-1
  Product1 : Product
  S1(t) : Product
  S2(t) : Product
  DSBSC : Outport
  wires:
  Product1/1 -> Add1/1
  Add/1 -> S1(t)/1
  Constant3/1 -> -S2(t)/2
  Constant2/1 -> Add1/2
  S2(t)/1 -> -S2(t)/1
  Carrier Signal/1 -> S1(t)/2, S2(t)/1
  Constant/1 -> Add/2
  Add1/1 -> S2(t)/2
  Constant1/1 -> Product1/2
  -S2(t)/1 -> Add2/2
  S1(t)/1 -> Add2/1
  Input Signal/1 -> Product1/1, Add/1
  Add2/1 -> DSBSC/1

== system signal_tranmission/SSB Demod98/Balanced Modulator1 ==
  note: -S2(t)
  note: S1(t)
  note: -m(t)
  note: m(t)
  note: S2(t)
  note: S1(t)
  Input Signal : Inport
  Carrier Signal : Inport  Port=2
  -S2(t) : Product
  Add : Sum
  Add1 : Sum
  Add2 : Sum
  Constant : Constant
  Constant1 : Constant  Value=-1
  Constant2 : Constant
  Constant3 : Constant  Value=-1
  Product1 : Product
  S1(t) : Product
  S2(t) : Product
  DSBSC : Outport
  wires:
  Product1/1 -> Add1/1
  Add/1 -> S1(t)/1
  Constant3/1 -> -S2(t)/2
  Constant2/1 -> Add1/2
  S2(t)/1 -> -S2(t)/1
  Carrier Signal/1 -> S1(t)/2, S2(t)/1
  Constant/1 -> Add/2
  Add1/1 -> S2(t)/2
  Constant1/1 -> Product1/2
  -S2(t)/1 -> Add2/2
  S1(t)/1 -> Add2/1
  Input Signal/1 -> Product1/1, Add/1
  Add2/1 -> DSBSC/1

== system signal_tranmission/SSB Demod99/Balanced Modulator1 ==
  note: -S2(t)
  note: S1(t)
  note: -m(t)
  note: m(t)
  note: S2(t)
  note: S1(t)
  Input Signal : Inport
  Carrier Signal : Inport  Port=2
  -S2(t) : Product
  Add : Sum
  Add1 : Sum
  Add2 : Sum
  Constant : Constant
  Constant1 : Constant  Value=-1
  Constant2 : Constant
  Constant3 : Constant  Value=-1
  Product1 : Product
  S1(t) : Product
  S2(t) : Product
  DSBSC : Outport
  wires:
  Product1/1 -> Add1/1
  Add/1 -> S1(t)/1
  Constant3/1 -> -S2(t)/2
  Constant2/1 -> Add1/2
  S2(t)/1 -> -S2(t)/1
  Carrier Signal/1 -> S1(t)/2, S2(t)/1
  Constant/1 -> Add/2
  Add1/1 -> S2(t)/2
  Constant1/1 -> Product1/2
  -S2(t)/1 -> Add2/2
  S1(t)/1 -> Add2/1
  Input Signal/1 -> Product1/1, Add/1
  Add2/1 -> DSBSC/1

== system signal_tranmission/SSB Modulator/Balanced Modulator ==
  note: -S2(t)
  note: S1(t)
  note: -m(t)
  note: m(t)
  note: S2(t)
  note: S1(t)
  Input Signal : Inport
  Carrier Signal : Inport  Port=2
  -S2(t) : Product
  Add : Sum
  Add1 : Sum
  Add2 : Sum
  Constant : Constant
  Constant1 : Constant  Value=-1
  Constant2 : Constant
  Constant3 : Constant  Value=-1
  Product1 : Product
  S1(t) : Product
  S2(t) : Product
  DSBSC : Outport
  wires:
  Product1/1 -> Add1/1
  Add/1 -> S1(t)/1
  Constant3/1 -> -S2(t)/2
  Constant2/1 -> Add1/2
  S2(t)/1 -> -S2(t)/1
  Carrier Signal/1 -> S1(t)/2, S2(t)/1
  Constant/1 -> Add/2
  Add1/1 -> S2(t)/2
  Constant1/1 -> Product1/2
  -S2(t)/1 -> Add2/2
  S1(t)/1 -> Add2/1
  Input Signal/1 -> Product1/1, Add/1
  Add2/1 -> DSBSC/1

== system signal_tranmission/SSB Modulator1/Balanced Modulator ==
  note: -S2(t)
  note: S1(t)
  note: -m(t)
  note: m(t)
  note: S2(t)
  note: S1(t)
  Input Signal : Inport
  Carrier Signal : Inport  Port=2
  -S2(t) : Product
  Add : Sum
  Add1 : Sum
  Add2 : Sum
  Constant : Constant
  Constant1 : Constant  Value=-1
  Constant2 : Constant
  Constant3 : Constant  Value=-1
  Product1 : Product
  S1(t) : Product
  S2(t) : Product
  DSBSC : Outport
  wires:
  Product1/1 -> Add1/1
  Add/1 -> S1(t)/1
  Constant3/1 -> -S2(t)/2
  Constant2/1 -> Add1/2
  S2(t)/1 -> -S2(t)/1
  Carrier Signal/1 -> S1(t)/2, S2(t)/1
  Constant/1 -> Add/2
  Add1/1 -> S2(t)/2
  Constant1/1 -> Product1/2
  -S2(t)/1 -> Add2/2
  S1(t)/1 -> Add2/1
  Input Signal/1 -> Product1/1, Add/1
  Add2/1 -> DSBSC/1

== system signal_tranmission/SSB Modulator10/Balanced Modulator ==
  note: -S2(t)
  note: S1(t)
  note: -m(t)
  note: m(t)
  note: S2(t)
  note: S1(t)
  Input Signal : Inport
  Carrier Signal : Inport  Port=2
  -S2(t) : Product
  Add : Sum
  Add1 : Sum
  Add2 : Sum
  Constant : Constant
  Constant1 : Constant  Value=-1
  Constant2 : Constant
  Constant3 : Constant  Value=-1
  Product1 : Product
  S1(t) : Product
  S2(t) : Product
  DSBSC : Outport
  wires:
  Product1/1 -> Add1/1
  Add/1 -> S1(t)/1
  Constant3/1 -> -S2(t)/2
  Constant2/1 -> Add1/2
  S2(t)/1 -> -S2(t)/1
  Carrier Signal/1 -> S1(t)/2, S2(t)/1
  Constant/1 -> Add/2
  Add1/1 -> S2(t)/2
  Constant1/1 -> Product1/2
  -S2(t)/1 -> Add2/2
  S1(t)/1 -> Add2/1
  Input Signal/1 -> Product1/1, Add/1
  Add2/1 -> DSBSC/1

== system signal_tranmission/SSB Modulator11/Balanced Modulator ==
  note: -S2(t)
  note: S1(t)
  note: -m(t)
  note: m(t)
  note: S2(t)
  note: S1(t)
  Input Signal : Inport
  Carrier Signal : Inport  Port=2
  -S2(t) : Product
  Add : Sum
  Add1 : Sum
  Add2 : Sum
  Constant : Constant
  Constant1 : Constant  Value=-1
  Constant2 : Constant
  Constant3 : Constant  Value=-1
  Product1 : Product
  S1(t) : Product
  S2(t) : Product
  DSBSC : Outport
  wires:
  Product1/1 -> Add1/1
  Add/1 -> S1(t)/1
  Constant3/1 -> -S2(t)/2
  Constant2/1 -> Add1/2
  S2(t)/1 -> -S2(t)/1
  Carrier Signal/1 -> S1(t)/2, S2(t)/1
  Constant/1 -> Add/2
  Add1/1 -> S2(t)/2
  Constant1/1 -> Product1/2
  -S2(t)/1 -> Add2/2
  S1(t)/1 -> Add2/1
  Input Signal/1 -> Product1/1, Add/1
  Add2/1 -> DSBSC/1

== system signal_tranmission/SSB Modulator12/Balanced Modulator ==
  note: -S2(t)
  note: S1(t)
  note: -m(t)
  note: m(t)
  note: S2(t)
  note: S1(t)
  Input Signal : Inport
  Carrier Signal : Inport  Port=2
  -S2(t) : Product
  Add : Sum
  Add1 : Sum
  Add2 : Sum
  Constant : Constant
  Constant1 : Constant  Value=-1
  Constant2 : Constant
  Constant3 : Constant  Value=-1
  Product1 : Product
  S1(t) : Product
  S2(t) : Product
  DSBSC : Outport
  wires:
  Product1/1 -> Add1/1
  Add/1 -> S1(t)/1
  Constant3/1 -> -S2(t)/2
  Constant2/1 -> Add1/2
  S2(t)/1 -> -S2(t)/1
  Carrier Signal/1 -> S1(t)/2, S2(t)/1
  Constant/1 -> Add/2
  Add1/1 -> S2(t)/2
  Constant1/1 -> Product1/2
  -S2(t)/1 -> Add2/2
  S1(t)/1 -> Add2/1
  Input Signal/1 -> Product1/1, Add/1
  Add2/1 -> DSBSC/1

== system signal_tranmission/SSB Modulator13/Balanced Modulator ==
  note: -S2(t)
  note: S1(t)
  note: -m(t)
  note: m(t)
  note: S2(t)
  note: S1(t)
  Input Signal : Inport
  Carrier Signal : Inport  Port=2
  -S2(t) : Product
  Add : Sum
  Add1 : Sum
  Add2 : Sum
  Constant : Constant
  Constant1 : Constant  Value=-1
  Constant2 : Constant
  Constant3 : Constant  Value=-1
  Product1 : Product
  S1(t) : Product
  S2(t) : Product
  DSBSC : Outport
  wires:
  Product1/1 -> Add1/1
  Add/1 -> S1(t)/1
  Constant3/1 -> -S2(t)/2
  Constant2/1 -> Add1/2
  S2(t)/1 -> -S2(t)/1
  Carrier Signal/1 -> S1(t)/2, S2(t)/1
  Constant/1 -> Add/2
  Add1/1 -> S2(t)/2
  Constant1/1 -> Product1/2
  -S2(t)/1 -> Add2/2
  S1(t)/1 -> Add2/1
  Input Signal/1 -> Product1/1, Add/1
  Add2/1 -> DSBSC/1

== system signal_tranmission/SSB Modulator14/Balanced Modulator ==
  note: -S2(t)
  note: S1(t)
  note: -m(t)
  note: m(t)
  note: S2(t)
  note: S1(t)
  Input Signal : Inport
  Carrier Signal : Inport  Port=2
  -S2(t) : Product
  Add : Sum
  Add1 : Sum
  Add2 : Sum
  Constant : Constant
  Constant1 : Constant  Value=-1
  Constant2 : Constant
  Constant3 : Constant  Value=-1
  Product1 : Product
  S1(t) : Product
  S2(t) : Product
  DSBSC : Outport
  wires:
  Product1/1 -> Add1/1
  Add/1 -> S1(t)/1
  Constant3/1 -> -S2(t)/2
  Constant2/1 -> Add1/2
  S2(t)/1 -> -S2(t)/1
  Carrier Signal/1 -> S1(t)/2, S2(t)/1
  Constant/1 -> Add/2
  Add1/1 -> S2(t)/2
  Constant1/1 -> Product1/2
  -S2(t)/1 -> Add2/2
  S1(t)/1 -> Add2/1
  Input Signal/1 -> Product1/1, Add/1
  Add2/1 -> DSBSC/1

== system signal_tranmission/SSB Modulator15/Balanced Modulator ==
  note: -S2(t)
  note: S1(t)
  note: -m(t)
  note: m(t)
  note: S2(t)
  note: S1(t)
  Input Signal : Inport
  Carrier Signal : Inport  Port=2
  -S2(t) : Product
  Add : Sum
  Add1 : Sum
  Add2 : Sum
  Constant : Constant
  Constant1 : Constant  Value=-1
  Constant2 : Constant
  Constant3 : Constant  Value=-1
  Product1 : Product
  S1(t) : Product
  S2(t) : Product
  DSBSC : Outport
  wires:
  Product1/1 -> Add1/1
  Add/1 -> S1(t)/1
  Constant3/1 -> -S2(t)/2
  Constant2/1 -> Add1/2
  S2(t)/1 -> -S2(t)/1
  Carrier Signal/1 -> S1(t)/2, S2(t)/1
  Constant/1 -> Add/2
  Add1/1 -> S2(t)/2
  Constant1/1 -> Product1/2
  -S2(t)/1 -> Add2/2
  S1(t)/1 -> Add2/1
  Input Signal/1 -> Product1/1, Add/1
  Add2/1 -> DSBSC/1

== system signal_tranmission/SSB Modulator16/Balanced Modulator ==
  note: -S2(t)
  note: S1(t)
  note: -m(t)
  note: m(t)
  note: S2(t)
  note: S1(t)
  Input Signal : Inport
  Carrier Signal : Inport  Port=2
  -S2(t) : Product
  Add : Sum
  Add1 : Sum
  Add2 : Sum
  Constant : Constant
  Constant1 : Constant  Value=-1
  Constant2 : Constant
  Constant3 : Constant  Value=-1
  Product1 : Product
  S1(t) : Product
  S2(t) : Product
  DSBSC : Outport
  wires:
  Product1/1 -> Add1/1
  Add/1 -> S1(t)/1
  Constant3/1 -> -S2(t)/2
  Constant2/1 -> Add1/2
  S2(t)/1 -> -S2(t)/1
  Carrier Signal/1 -> S1(t)/2, S2(t)/1
  Constant/1 -> Add/2
  Add1/1 -> S2(t)/2
  Constant1/1 -> Product1/2
  -S2(t)/1 -> Add2/2
  S1(t)/1 -> Add2/1
  Input Signal/1 -> Product1/1, Add/1
  Add2/1 -> DSBSC/1

== system signal_tranmission/SSB Modulator17/Balanced Modulator ==
  note: -S2(t)
  note: S1(t)
  note: -m(t)
  note: m(t)
  note: S2(t)
  note: S1(t)
  Input Signal : Inport
  Carrier Signal : Inport  Port=2
  -S2(t) : Product
  Add : Sum
  Add1 : Sum
  Add2 : Sum
  Constant : Constant
  Constant1 : Constant  Value=-1
  Constant2 : Constant
  Constant3 : Constant  Value=-1
  Product1 : Product
  S1(t) : Product
  S2(t) : Product
  DSBSC : Outport
  wires:
  Product1/1 -> Add1/1
  Add/1 -> S1(t)/1
  Constant3/1 -> -S2(t)/2
  Constant2/1 -> Add1/2
  S2(t)/1 -> -S2(t)/1
  Carrier Signal/1 -> S1(t)/2, S2(t)/1
  Constant/1 -> Add/2
  Add1/1 -> S2(t)/2
  Constant1/1 -> Product1/2
  -S2(t)/1 -> Add2/2
  S1(t)/1 -> Add2/1
  Input Signal/1 -> Product1/1, Add/1
  Add2/1 -> DSBSC/1

== system signal_tranmission/SSB Modulator18/Balanced Modulator ==
  note: -S2(t)
  note: S1(t)
  note: -m(t)
  note: m(t)
  note: S2(t)
  note: S1(t)
  Input Signal : Inport
  Carrier Signal : Inport  Port=2
  -S2(t) : Product
  Add : Sum
  Add1 : Sum
  Add2 : Sum
  Constant : Constant
  Constant1 : Constant  Value=-1
  Constant2 : Constant
  Constant3 : Constant  Value=-1
  Product1 : Product
  S1(t) : Product
  S2(t) : Product
  DSBSC : Outport
  wires:
  Product1/1 -> Add1/1
  Add/1 -> S1(t)/1
  Constant3/1 -> -S2(t)/2
  Constant2/1 -> Add1/2
  S2(t)/1 -> -S2(t)/1
  Carrier Signal/1 -> S1(t)/2, S2(t)/1
  Constant/1 -> Add/2
  Add1/1 -> S2(t)/2
  Constant1/1 -> Product1/2
  -S2(t)/1 -> Add2/2
  S1(t)/1 -> Add2/1
  Input Signal/1 -> Product1/1, Add/1
  Add2/1 -> DSBSC/1

== system signal_tranmission/SSB Modulator19/Balanced Modulator ==
  note: -S2(t)
  note: S1(t)
  note: -m(t)
  note: m(t)
  note: S2(t)
  note: S1(t)
  Input Signal : Inport
  Carrier Signal : Inport  Port=2
  -S2(t) : Product
  Add : Sum
  Add1 : Sum
  Add2 : Sum
  Constant : Constant
  Constant1 : Constant  Value=-1
  Constant2 : Constant
  Constant3 : Constant  Value=-1
  Product1 : Product
  S1(t) : Product
  S2(t) : Product
  DSBSC : Outport
  wires:
  Product1/1 -> Add1/1
  Add/1 -> S1(t)/1
  Constant3/1 -> -S2(t)/2
  Constant2/1 -> Add1/2
  S2(t)/1 -> -S2(t)/1
  Carrier Signal/1 -> S1(t)/2, S2(t)/1
  Constant/1 -> Add/2
  Add1/1 -> S2(t)/2
  Constant1/1 -> Product1/2
  -S2(t)/1 -> Add2/2
  S1(t)/1 -> Add2/1
  Input Signal/1 -> Product1/1, Add/1
  Add2/1 -> DSBSC/1

== system signal_tranmission/SSB Modulator2/Balanced Modulator ==
  note: -S2(t)
  note: S1(t)
  note: -m(t)
  note: m(t)
  note: S2(t)
  note: S1(t)
  Input Signal : Inport
  Carrier Signal : Inport  Port=2
  -S2(t) : Product
  Add : Sum
  Add1 : Sum
  Add2 : Sum
  Constant : Constant
  Constant1 : Constant  Value=-1
  Constant2 : Constant
  Constant3 : Constant  Value=-1
  Product1 : Product
  S1(t) : Product
  S2(t) : Product
  DSBSC : Outport
  wires:
  Product1/1 -> Add1/1
  Add/1 -> S1(t)/1
  Constant3/1 -> -S2(t)/2
  Constant2/1 -> Add1/2
  S2(t)/1 -> -S2(t)/1
  Carrier Signal/1 -> S1(t)/2, S2(t)/1
  Constant/1 -> Add/2
  Add1/1 -> S2(t)/2
  Constant1/1 -> Product1/2
  -S2(t)/1 -> Add2/2
  S1(t)/1 -> Add2/1
  Input Signal/1 -> Product1/1, Add/1
  Add2/1 -> DSBSC/1

== system signal_tranmission/SSB Modulator20/Balanced Modulator ==
  note: -S2(t)
  note: S1(t)
  note: -m(t)
  note: m(t)
  note: S2(t)
  note: S1(t)
  Input Signal : Inport
  Carrier Signal : Inport  Port=2
  -S2(t) : Product
  Add : Sum
  Add1 : Sum
  Add2 : Sum
  Constant : Constant
  Constant1 : Constant  Value=-1
  Constant2 : Constant
  Constant3 : Constant  Value=-1
  Product1 : Product
  S1(t) : Product
  S2(t) : Product
  DSBSC : Outport
  wires:
  Product1/1 -> Add1/1
  Add/1 -> S1(t)/1
  Constant3/1 -> -S2(t)/2
  Constant2/1 -> Add1/2
  S2(t)/1 -> -S2(t)/1
  Carrier Signal/1 -> S1(t)/2, S2(t)/1
  Constant/1 -> Add/2
  Add1/1 -> S2(t)/2
  Constant1/1 -> Product1/2
  -S2(t)/1 -> Add2/2
  S1(t)/1 -> Add2/1
  Input Signal/1 -> Product1/1, Add/1
  Add2/1 -> DSBSC/1
